simulink model "jeb_ut"  (Simulink 8.1)
settings: Solver=FixedStepDiscrete  StartTime=0.0  StopTime=10  FixedStep=5E-3  RelTol=1e-3
PostLoadFcn:
  | , if any(exist('dsrtsu_mdlpostloadfcn', 'file') == [2, 3, 6]), try dsrtsu_mdlpostloadfcn('Execute', bdroot); catch fprintf('Error in PostLoadFcn (dsrtsu_mdlpostloadfcn) for model "%s":\n %s\n', bdroot, lasterr); end, end,
undefined symbols (not defined in the file or in its folder): VDHP_DisableADASFun_flg, VDHP_DisableAEB_flg, VDINR_AEBEnableH_flg, VDINR_AEBEnableO_flg, VDINR_HMICANValid_flg, VDINR_KeySwitchStatus_enum, VDINR_VehSpd_kph, VDINR_VehSpd_mps, VPER_CameraStatus_enum, VPER_FusionStatus_enum, VPER_RadarStatus_enum
libraries: siltestlib x33, jeb x1
settings Model: DSRTSU_INTERNAL_RTI_VER=450  DSRTSU_INTERNAL_RTI_TYPE=rti1401  RTICANMMDATA=struct('GeneralSetupData',struct('modelroot','D:\ELN150201_TAIWAN\trunk\AdasDragon\software\sw_development\arch\app\jud','generalsettings',struct('filesettings',struct('destfolder',struct('Name','RTICANMM_FILES','Check',1),'buildfolder',struct('Name','.','Check',1),'AbsDestfolder',struct('Name','D:\ELN150201_TAIWAN\trunk\AdasDragon\software\sw_development\arch\app\jud\RTICANMM_FILES'),'AbsBuildfolder',struct('Name','D:\ELN150201_TAIWAN\trunk\AdasDragon\software\sw_development\arch\app\jud'))),'options',struct('addpaths',1,'rmpaths',1,'addtrcexclusion',logical(1),'cannavigator',struct('checkmonitoring',0),'show_usrtrc',0,'use_usrtrc',0),'advanced',struct('options',[1 1 1 1 1 1 1 1 1 1 1 1 1 1 1 1 1 1 1 1 1 1 1 1 1 1 1 1 1 1 1 1 1 1 1 1 1 1 1 1 1 1 1 1 1 1 1 1 1 1 1 1 1 1 1 1 1 1 1 1 1 1 1 1 1 1 1 1 1 1 1 1 1 1 1 1 1 1 1 1 1 1 1 1 1 1 1 1 1 1 1 1 1 1 1 1 1 1 1 1]),'MPSetup',{{}},'modelname','jeb_ut','block','jeb_ut'))  DSRTSU_INTERNAL_RTIFPGA=40  Creator=AT015411  LastModifiedBy=AT015555  BufferReuse=off
settings DataIOCC: SignalLoggingSaveFormat=Dataset
settings OptimizationCC: BlockReduction=off  OptimizeBlockIOStorage=off  BufferReuse=off  ExpressionFolding=off  ExpressionDepthLimit=128  LocalBlockOutputs=off
settings DebuggingCC: FcnCallInpInsideContextMsg=EnableAllAsError
settings HardwareCC: ProdIntDivRoundTo=Zero  ProdEndianess=BigEndian  ProdHWDeviceType=Generic->Custom  TargetIntDivRoundTo=Zero  TargetEndianess=BigEndian  TargetHWDeviceType=Generic->Custom
settings RTWCC: SystemTargetFile=rti1005.tlc  MakeCommand=make_rti  TemplateMakefile=rti1005.tmf  Description=dSPACE DS1005 Hardware Platform  ProcessScript=rti1005_make_rtw_hook
settings STFCustomTargetCC: CodeReplacementLibrary=ANSI_C  ParMdlRefBuildCompliant=on  GeneratePreprocessorConditionals=Disable all  MatFileLogging=on  SystemTargetFile=rti1005.tlc
settings GRTTargetCC: CompOptLevelCompliant=off  ConcurrentExecutionCompliant=off  ExtModeMexFile=noextcomm
settings CustomProperty: DataType=RTWOptions_EnumType_C__Program Files (x86)_dSPACE RCPHIL 2014-B_MATLAB_RTI_RTI1401_TLC_rti1005_1InitialSimState  Value=RUN
settings EnumStrPairs: String=RUN

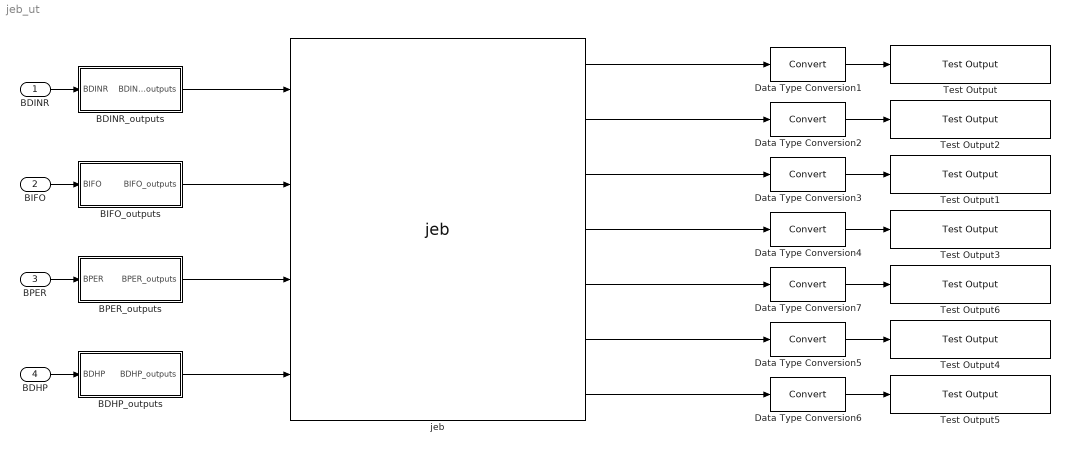
== system jeb_ut ==
  BDINR : Inport  OutDataTypeStr=Bus: BDINR_outputs
  BIFO : Inport  Port=2  OutDataTypeStr=Bus: BIFO_outputs
  BPER : Inport  Port=3  OutDataTypeStr=Bus: BPER_outputs
  BDHP : Inport  Port=4  OutDataTypeStr=Bus: BDHP_outputs
  BDHP_outputs : Subsystem
  BDINR_outputs : Subsystem
  BIFO_outputs : Subsystem
  BPER_outputs : Subsystem
  Data Type Conversion{1..7} (7 alike) : DataTypeConversion
  Test Output : siltestlib/Test Output  varname=VJUD_AEBEnableReq_flg  sampletime=-1
  Test Output1 : siltestlib/Test Output  varname=VJUD_AEBSpeedInRange_flg  sampletime=-1
  Test Output2 : siltestlib/Test Output  varname=VJUD_AEBOperational_flg  sampletime=-1
  Test Output3 : siltestlib/Test Output  varname=VJUD_AEBActingReq_flg  sampletime=-1
  Test Output4 : siltestlib/Test Output  varname=VJUD_AEBAutoBraking_flg  sampletime=-1
  Test Output5 : siltestlib/Test Output  varname=VJUD_AEBDeactivationReq_flg  sampletime=-1
  Test Output6 : siltestlib/Test Output  varname=VJUD_AEBReturnOperational_flg  sampletime=-1
  jeb : jeb/jeb
  wires:
  BDINR_outputs/1(BDINR_outputs) -> jeb/1
  BIFO_outputs/1(BIFO_outputs) -> jeb/2
  BPER_outputs/1(BPER_outputs) -> jeb/3
  BDINR/1 -> BDINR_outputs/1(BDINR)
  BPER/1 -> BPER_outputs/1(BPER)
  BIFO/1 -> BIFO_outputs/1(BIFO)
  BDHP_outputs/1(BDHP_outputs) -> jeb/4
  BDHP/1 -> BDHP_outputs/1(BDHP)
  Data Type Conversion1/1 -> Test Output/1
  Data Type Conversion2/1 -> Test Output2/1
  Data Type Conversion3/1 -> Test Output1/1
  Data Type Conversion4/1 -> Test Output3/1
  Data Type Conversion5/1 -> Test Output4/1
  Data Type Conversion6/1 -> Test Output5/1
  jeb/1 -> Data Type Conversion1/1
  jeb/2 -> Data Type Conversion2/1
  jeb/3 -> Data Type Conversion3/1
  jeb/4 -> Data Type Conversion4/1
  jeb/6 -> Data Type Conversion5/1
  jeb/7 -> Data Type Conversion6/1
  Data Type Conversion7/1 -> Test Output6/1
  jeb/5 -> Data Type Conversion7/1

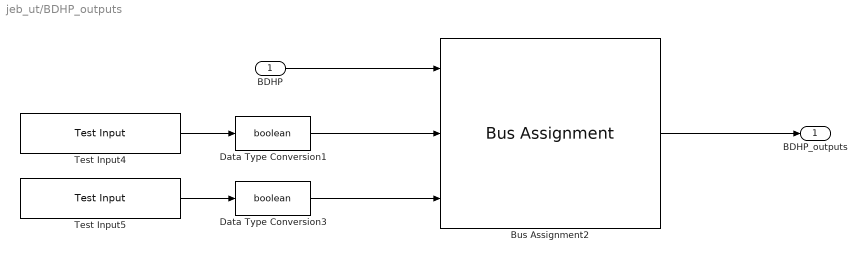
== system jeb_ut/BDHP_outputs ==
  BDHP : Inport  OutDataTypeStr=Bus: BDHP_outputs
  Bus Assignment2 : BusAssignment  AssignedSignals=VDHP_DisableADASFun_flg,VDHP_DisableAEB_flg
  Data Type Conversion1 : DataTypeConversion  OutDataTypeStr=boolean
  Data Type Conversion3 : DataTypeConversion  OutDataTypeStr=boolean
  Test Input4 : siltestlib/Test Input  varname=VDHP_DisableADASFun_flg  sampletime=-1
  Test Input5 : siltestlib/Test Input  varname=VDHP_DisableAEB_flg  sampletime=-1
  BDHP_outputs : Outport  OutDataTypeStr=Bus: BDHP_outputs
  wires:
  BDHP/1 -> Bus Assignment2/1
  Bus Assignment2/1 -> BDHP_outputs/1
  Test Input4/1 -> Data Type Conversion1/1
  Data Type Conversion1/1 -> Bus Assignment2/2
  Test Input5/1 -> Data Type Conversion3/1
  Data Type Conversion3/1 -> Bus Assignment2/3

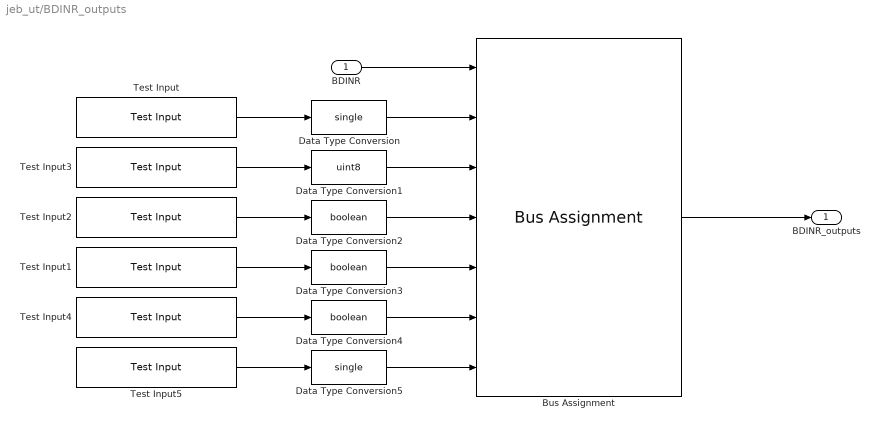
== system jeb_ut/BDINR_outputs ==
  BDINR : Inport  OutDataTypeStr=Bus: BDINR_outputs
  Bus Assignment : BusAssignment  AssignedSignals=VDINR_VehSpd_kph,VDINR_KeySwitchStatus_enum,VDINR_HMICANValid_flg,VDINR_AEBEnableH_flg,VDINR_AEBEnableO_flg,VDINR_VehSpd_mps
  Data Type Conversion : DataTypeConversion  OutDataTypeStr=single
  Data Type Conversion1 : DataTypeConversion  OutDataTypeStr=uint8
  Data Type Conversion2 : DataTypeConversion  OutDataTypeStr=boolean
  Data Type Conversion3 : DataTypeConversion  OutDataTypeStr=boolean
  Data Type Conversion4 : DataTypeConversion  OutDataTypeStr=boolean
  Data Type Conversion5 : DataTypeConversion  OutDataTypeStr=single
  Test Input : siltestlib/Test Input  varname=VDINR_VehSpd_kph  sampletime=-1
  Test Input1 : siltestlib/Test Input  varname=VDINR_AEBEnableH_flg  sampletime=-1
  Test Input2 : siltestlib/Test Input  varname=VDINR_HMICANValid_flg  sampletime=-1
  Test Input3 : siltestlib/Test Input  varname=VDINR_KeySwitchStatus_enum  sampletime=-1
  Test Input4 : siltestlib/Test Input  varname=VDINR_AEBEnableO_flg  sampletime=-1
  Test Input5 : siltestlib/Test Input  varname=VDINR_VehSpd_mps  sampletime=-1
  BDINR_outputs : Outport  OutDataTypeStr=Bus: BDINR_outputs
  wires:
  Bus Assignment/1 -> BDINR_outputs/1
  BDINR/1 -> Bus Assignment/1
  Test Input/1 -> Data Type Conversion/1
  Data Type Conversion/1 -> Bus Assignment/2
  Test Input3/1 -> Data Type Conversion1/1
  Data Type Conversion1/1 -> Bus Assignment/3
  Test Input2/1 -> Data Type Conversion2/1
  Data Type Conversion2/1 -> Bus Assignment/4
  Test Input1/1 -> Data Type Conversion3/1
  Data Type Conversion3/1 -> Bus Assignment/5
  Test Input4/1 -> Data Type Conversion4/1
  Data Type Conversion4/1 -> Bus Assignment/6
  Test Input5/1 -> Data Type Conversion5/1
  Data Type Conversion5/1 -> Bus Assignment/7

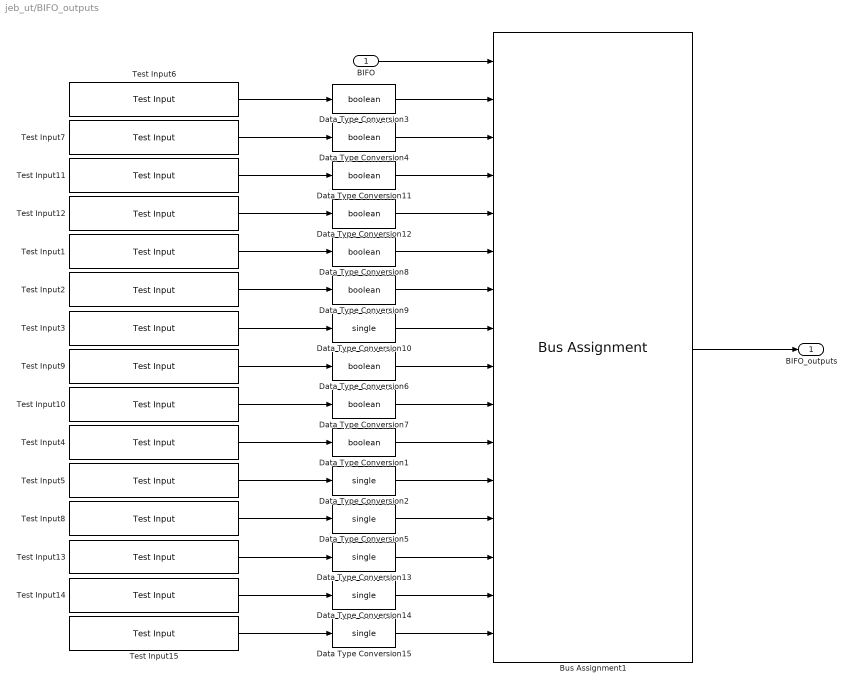
== system jeb_ut/BIFO_outputs ==
  BIFO : Inport  OutDataTypeStr=Bus: BIFO_outputs
  Bus Assignment1 : BusAssignment  AssignedSignals=VIFO_ParkingSituation_flg,VIFO_DriverOverrideReq_flg,VIFO_AEBTargetVehAssigned_flg,VIFO_VRUTargetPedAssigned_flg,VIFO_AggressiveDriverDetec_flg,VIFO_ActiveDriverDetec_flg,VIFO_AEBTargetVehRelSpeedX_mps,VIFO_VehicleStatusOk_flg,VIFO_DriverSafetyStatusOk_flg,VIFO_BrakePedalPressed_flg,VIFO_AEBVehClearance_m,VIFO_AEBMCLongAcc_mps2,VIFO_VRUTargetPedRelSpeedX_mps,VIFO_VRUPedClearance_m,VIFO_AEBTGap_s
  Data Type Conversion{1,3..4,6..9,11..12} (9 alike) : DataTypeConversion  OutDataTypeStr=boolean
  Data Type Conversion{2,5,10,13..15} (6 alike) : DataTypeConversion  OutDataTypeStr=single
  Test Input1 : siltestlib/Test Input  varname=VIFO_AggressiveDriverDetec_flg  sampletime=-1
  Test Input10 : siltestlib/Test Input  varname=VIFO_DriverSafetyStatusOk_flg  sampletime=-1
  Test Input11 : siltestlib/Test Input  varname=VIFO_AEBTargetVehAssigned_flg  sampletime=-1
  Test Input12 : siltestlib/Test Input  varname=VIFO_VRUTargetPedAssigned_flg  sampletime=-1
  Test Input13 : siltestlib/Test Input  varname=VIFO_VRUTargetPedRelSpeedX_mps  sampletime=-1
  Test Input14 : siltestlib/Test Input  varname=VIFO_VRUPedClearance_m  sampletime=-1
  Test Input15 : siltestlib/Test Input  varname=VIFO_AEBTGap_s  sampletime=-1
  Test Input2 : siltestlib/Test Input  varname=VIFO_ActiveDriverDetec_flg  sampletime=-1
  Test Input3 : siltestlib/Test Input  varname=VIFO_AEBTargetVehRelSpeedX_mps  sampletime=-1
  Test Input4 : siltestlib/Test Input  varname=VIFO_BrakePedalPressed_flg  sampletime=-1
  Test Input5 : siltestlib/Test Input  varname=VIFO_AEBVehClearance_m  sampletime=-1
  Test Input6 : siltestlib/Test Input  varname=VIFO_ParkingSituation_flg  sampletime=-1
  Test Input7 : siltestlib/Test Input  varname=VIFO_DriverOverrideReq_flg  sampletime=-1
  Test Input8 : siltestlib/Test Input  varname=VIFO_AEBMCLongAcc_mps2  sampletime=-1
  Test Input9 : siltestlib/Test Input  varname=VIFO_VehicleStatusOk_flg  sampletime=-1
  BIFO_outputs : Outport  OutDataTypeStr=Bus: BIFO_outputs
  wires:
  BIFO/1 -> Bus Assignment1/1
  Bus Assignment1/1 -> BIFO_outputs/1
  Test Input1/1 -> Data Type Conversion8/1
  Test Input2/1 -> Data Type Conversion9/1
  Test Input3/1 -> Data Type Conversion10/1
  Test Input4/1 -> Data Type Conversion1/1
  Test Input5/1 -> Data Type Conversion2/1
  Test Input6/1 -> Data Type Conversion3/1
  Test Input7/1 -> Data Type Conversion4/1
  Test Input9/1 -> Data Type Conversion6/1
  Test Input10/1 -> Data Type Conversion7/1
  Data Type Conversion4/1 -> Bus Assignment1/3
  Data Type Conversion3/1 -> Bus Assignment1/2
  Data Type Conversion8/1 -> Bus Assignment1/6
  Data Type Conversion9/1 -> Bus Assignment1/7
  Test Input11/1 -> Data Type Conversion11/1
  Test Input12/1 -> Data Type Conversion12/1
  Data Type Conversion11/1 -> Bus Assignment1/4
  Data Type Conversion12/1 -> Bus Assignment1/5
  Data Type Conversion10/1 -> Bus Assignment1/8
  Data Type Conversion6/1 -> Bus Assignment1/9
  Data Type Conversion7/1 -> Bus Assignment1/10
  Data Type Conversion1/1 -> Bus Assignment1/11
  Data Type Conversion2/1 -> Bus Assignment1/12
  Test Input8/1 -> Data Type Conversion5/1
  Data Type Conversion5/1 -> Bus Assignment1/13
  Test Input13/1 -> Data Type Conversion13/1
  Data Type Conversion13/1 -> Bus Assignment1/14
  Test Input14/1 -> Data Type Conversion14/1
  Data Type Conversion14/1 -> Bus Assignment1/15
  Test Input15/1 -> Data Type Conversion15/1
  Data Type Conversion15/1 -> Bus Assignment1/16

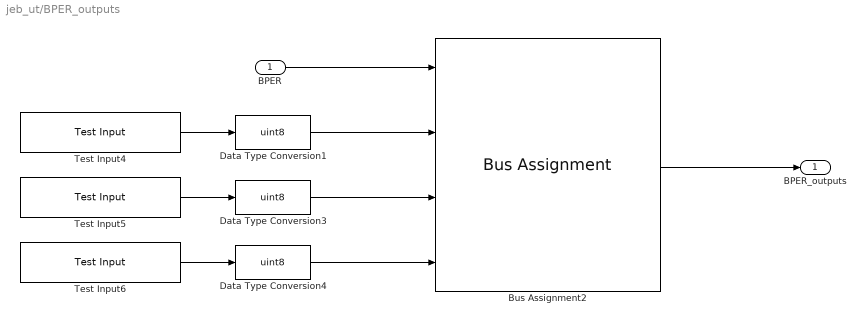
== system jeb_ut/BPER_outputs ==
  BPER : Inport  OutDataTypeStr=Bus: BPER_outputs
  Bus Assignment2 : BusAssignment  AssignedSignals=VPER_CameraStatus_enum,VPER_RadarStatus_enum,VPER_FusionStatus_enum
  Data Type Conversion1 : DataTypeConversion  OutDataTypeStr=uint8
  Data Type Conversion3 : DataTypeConversion  OutDataTypeStr=uint8
  Data Type Conversion4 : DataTypeConversion  OutDataTypeStr=uint8
  Test Input4 : siltestlib/Test Input  varname=VPER_CameraStatus_enum  sampletime=-1
  Test Input5 : siltestlib/Test Input  varname=VPER_RadarStatus_enum  sampletime=-1
  Test Input6 : siltestlib/Test Input  varname=VPER_FusionStatus_enum  sampletime=-1
  BPER_outputs : Outport  OutDataTypeStr=Bus: BPER_outputs
  wires:
  BPER/1 -> Bus Assignment2/1
  Bus Assignment2/1 -> BPER_outputs/1
  Test Input4/1 -> Data Type Conversion1/1
  Data Type Conversion1/1 -> Bus Assignment2/2
  Test Input5/1 -> Data Type Conversion3/1
  Data Type Conversion3/1 -> Bus Assignment2/3
  Test Input6/1 -> Data Type Conversion4/1
  Data Type Conversion4/1 -> Bus Assignment2/4
